simulink model "untitled1111111"  (R2018b)
settings: Solver=FixedStepDiscrete  StartTime=0.0  StopTime=Inf  RelTol=1e-3  EnableMultiTasking=on
undefined symbols (not defined in the file or in its folder): radians
libraries: c2837xDlib x4, tiiqmathlib x3
settings Model: ExtModeTrigDuration=8  Creator=mocan  LastModifiedBy=mocan
settings OptimizationCC: DefaultUnderspecifiedDataType=single  EnhancedBackFolding=on  PassReuseOutputArgsAs=Individual arguments  MaxStackSize=512  OptimizeBlockOrder=speed  DifferentSizesBufferReuse=on  OptimizationCustomize=off
settings DebuggingCC: ParameterPrecisionLossMsg=none  ParameterTunabilityLossMsg=error
settings HardwareCC: ProdBitPerChar=16  ProdBitPerInt=16  ProdBitPerPointer=32  ProdBitPerSizeT=32  ProdBitPerPtrDiffT=32  ProdLargestAtomicInteger=Integer  ProdLargestAtomicFloat=None  ProdWordSize=16  ProdLongLongMode=on  ProdHWDeviceType=Texas Instruments->C2000
settings SFSimCC: MATLABDynamicMemAlloc=off
settings RTWCC: SystemTargetFile=ert.tlc  HardwareBoard=TI Delfino F2837xD  TemplateMakefile=ert_default_tmf  GenerateReport=on  Toolchain=Texas Instruments Code Composer Studio (C2000)  IncludeHyperlinkInReport=on  LaunchReport=on  GenerateTraceInfo=on  GenerateTraceReport=on  GenerateTraceReportSl=on  GenerateTraceReportSf=on  GenerateTraceReportEml=on
settings CodeAppCC: ForceParamTrailComments=on  IgnoreCustomStorageClasses=off  OperatorAnnotations=on  SimulinkDataObjDesc=on  SFDataObjDesc=on  InsertBlockDesc=on
settings ERTTargetCC: CodeReplacementLibrary=TI C28x

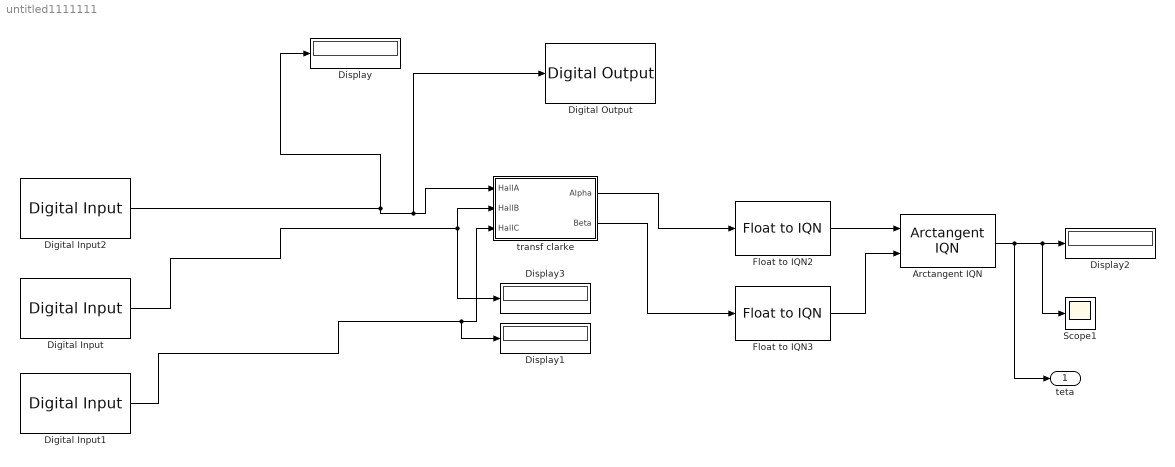
== system untitled1111111 ==
  Arctangent IQN : tiiqmathlib/Arctangent IQN  tanOption=atan2 (radians)
      settings: SourceProductBaseCode=TIC2000
  Digital Input : c2837xDlib/Digital Input  GPIO_Number=GPIO24~GPIO31  GPIO_Bit0=off  GPIO_Bit1=off  GPIO_Bit2=on  GPIO_Bit3=off  GPIO_Bit4=off  GPIO_Bit5=off  GPIO_Bit6=off  GPIO_Bit7=off  sampleTime=0.1  dataType=auto  GPIO_Bit0_Qualification=Sync to SYSCLKOUT  GPIO_Bit1_Qualification=Sync to SYSCLKOUT  GPIO_Bit2_Qualification=Sync to SYSCLKOUT  GPIO_Bit3_Qualification=Sync to SYSCLKOUT  GPIO_Bit4_Qualification=Sync to SYSCLKOUT  GPIO_Bit5_Qualification=Sync to SYSCLKOUT  GPIO_Bit6_Qualification=Sync to SYSCLKOUT  GPIO_Bit7_Qualification=Sync to SYSCLKOUT  Qualification_Period=-1
      settings: SourceProductBaseCode=TIC2000
  Digital Input1 : c2837xDlib/Digital Input  GPIO_Number=GPIO24~GPIO31  GPIO_Bit0=off  GPIO_Bit1=off  GPIO_Bit2=off  GPIO_Bit3=on  GPIO_Bit4=off  GPIO_Bit5=off  GPIO_Bit6=off  GPIO_Bit7=off  sampleTime=0.1  dataType=auto  GPIO_Bit0_Qualification=Sync to SYSCLKOUT  GPIO_Bit1_Qualification=Sync to SYSCLKOUT  GPIO_Bit2_Qualification=Sync to SYSCLKOUT  GPIO_Bit3_Qualification=Sync to SYSCLKOUT  GPIO_Bit4_Qualification=Sync to SYSCLKOUT  GPIO_Bit5_Qualification=Sync to SYSCLKOUT  GPIO_Bit6_Qualification=Sync to SYSCLKOUT  GPIO_Bit7_Qualification=Sync to SYSCLKOUT  Qualification_Period=-1
      settings: SourceProductBaseCode=TIC2000
  Digital Input2 : c2837xDlib/Digital Input  GPIO_Number=GPIO24~GPIO31  GPIO_Bit0=off  GPIO_Bit1=on  GPIO_Bit2=off  GPIO_Bit3=off  GPIO_Bit4=off  GPIO_Bit5=off  GPIO_Bit6=off  GPIO_Bit7=off  sampleTime=0.1  dataType=auto  GPIO_Bit0_Qualification=Sync to SYSCLKOUT  GPIO_Bit1_Qualification=Sync to SYSCLKOUT  GPIO_Bit2_Qualification=Sync to SYSCLKOUT  GPIO_Bit3_Qualification=Sync to SYSCLKOUT  GPIO_Bit4_Qualification=Sync to SYSCLKOUT  GPIO_Bit5_Qualification=Sync to SYSCLKOUT  GPIO_Bit6_Qualification=Sync to SYSCLKOUT  GPIO_Bit7_Qualification=Sync to SYSCLKOUT  Qualification_Period=-1
      settings: SourceProductBaseCode=TIC2000
  Digital Output : c2837xDlib/Digital Output  GPIO_Number=GPIO32~GPIO39  GPIO_Bit0=off  GPIO_BIT0_Toggle=off  GPIO_Bit1=off  GPIO_BIT1_Toggle=off  GPIO_Bit2=on  GPIO_BIT2_Toggle=off  GPIO_Bit3=off  GPIO_BIT3_Toggle=off  GPIO_Bit4=off  GPIO_BIT4_Toggle=off  GPIO_Bit5=off  GPIO_BIT5_Toggle=off  GPIO_Bit6=off  GPIO_BIT6_Toggle=off  GPIO_Bit7=off  GPIO_BIT7_Toggle=off
      settings: SourceProductName=Embedded Coder Support Package for Texas Instruments C2000 Processors  SourceProductBaseCode=TIC2000
  Display{,1..3} (4 alike) : Display
  Float to IQN2 : tiiqmathlib/Float to IQN  Q_value=28
      settings: SourceProductBaseCode=TIC2000
  Float to IQN3 : tiiqmathlib/Float to IQN  Q_value=28
      settings: SourceProductBaseCode=TIC2000
  Scope1 : Scope
  transf clarke : Subsystem
  teta : Outport  VectorParamsAs1DForOutWhenUnconnected=on
  wires:
  Digital Input1/1 -> transf clarke/3(HallC), Display1/1
  Float to IQN2/1 -> Arctangent IQN/1
  Arctangent IQN/1 -> Display2/1, Scope1/1, teta/1
  Float to IQN3/1 -> Arctangent IQN/2
  transf clarke/1(Alpha) -> Float to IQN2/1
  Digital Input2/1 -> Digital Output/1, transf clarke/1(HallA), Display/1
  transf clarke/2(Beta) -> Float to IQN3/1
  Digital Input/1 -> transf clarke/2(HallB), Display3/1

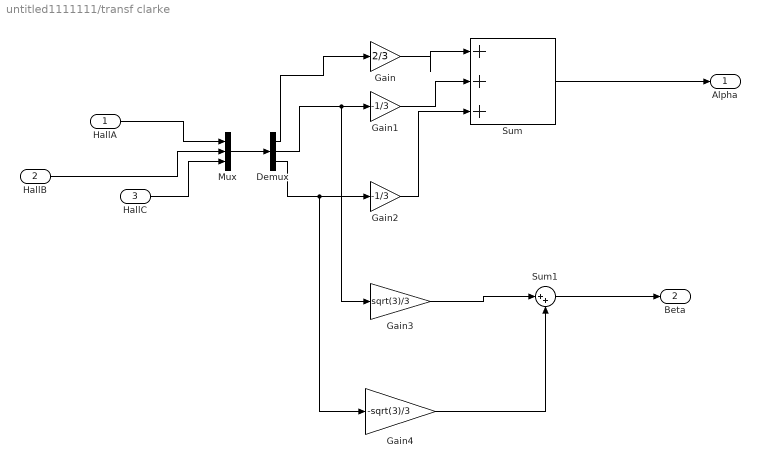
== system untitled1111111/transf clarke ==
  HallA : Inport
  HallB : Inport  Port=2
  HallC : Inport  Port=3
  Demux : Demux  Outputs=3
  Gain : Gain  Gain=2/3
  Gain1 : Gain  Gain=-1/3
  Gain2 : Gain  Gain=-1/3
  Gain3 : Gain  Gain=sqrt(3)/3
  Gain4 : Gain  Gain=-sqrt(3)/3
  Mux : Mux  Inputs=3
  Sum : Sum  Inputs=|+++  OutDataTypeStr=single
  Sum1 : Sum  Inputs=|++  AccumDataTypeStr=single
  Alpha : Outport  VectorParamsAs1DForOutWhenUnconnected=on
  Beta : Outport  Port=2  VectorParamsAs1DForOutWhenUnconnected=on
  wires:
  Mux/1 -> Demux/1
  HallC/1 -> Mux/3
  HallB/1 -> Mux/2
  HallA/1 -> Mux/1
  Gain3/1 -> Sum1/1
  Gain4/1 -> Sum1/2
  Gain2/1 -> Sum/3
  Sum1/1 -> Beta/1
  Gain1/1 -> Sum/2
  Sum/1 -> Alpha/1
  Demux/3 -> Gain2/1, Gain4/1
  Gain/1 -> Sum/1
  Demux/2 -> Gain1/1, Gain3/1
  Demux/1 -> Gain/1
